simulink library "mbed_lib.tmp"  (R2015a)
settings: Solver=ode45  SolverMode=SingleTasking  StartTime=0.0  StopTime=10.0  RelTol=1e-3
undefined symbols (not defined in the file): A
libraries: mbed_lib x1
settings Model: CovSFcnEnable=off  Creator=syoon  LastModifiedBy=oh
settings OptimizationCC: BlockReduction=off  BooleanDataType=off
settings DebuggingCC: SaveWithParameterizedLinksMsg=none  UnderspecifiedInitializationDetection=Classic  MergeDetectMultiDrivingBlocksExec=none  SignalResolutionControl=TryResolveAllWithWarning  StrictBusMsg=Warning
settings HardwareCC: TargetUnknown=on

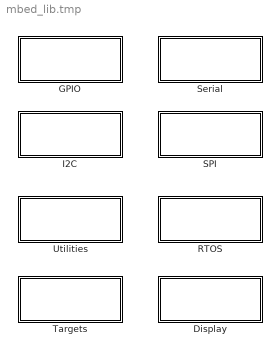
== system mbed_lib.tmp ==
  Display : Subsystem
      settings: OpenFcn=LCDScope
      mask Display: disp('Display')
  GPIO : Subsystem
      mask Display: disp('GPIO')
  I2C : Subsystem
      mask Display: disp('I2C')
  RTOS : Subsystem
      mask Display: disp('RTOS')
  SPI : Subsystem
      mask Display: disp('SPI')
  Serial : Subsystem
      mask Display: disp('Serial')
  Targets : Subsystem
      settings: OpenFcn=mbed_targets
      mask Display: disp('Targets')
  Utilities : Subsystem
      mask Display: disp('Utilities')

== system mbed_lib.tmp/Display ==

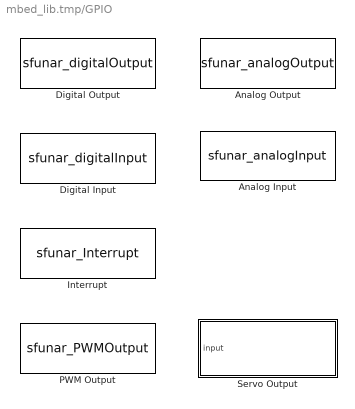
== system mbed_lib.tmp/GPIO ==
  Analog Input : S-Function  FunctionName=sfunar_analogInput  Parameters=uint8(SParameter1), SampleTime, uint8(SParameter2)  mask(mbed Analog Input){SParameter2=A, SParameter1=0, SampleTime=-1}
      mask prompts: SParameter2 "Port Name:"; SParameter1 "Pin Number:"; SampleTime "Sample time (-1 for inherited):"
      mask help:
      | Reads the analog voltage input from the specified pin.
      |
      | The range of input on the pin is between 0 and Vref corresponding to a block output of 0 to 1.0f (in %) or 0 to 1024/4096/.. .
      mask Help:
      | <p>This block calls the AnalogIn.read() and AnalogIn.read_u16() function from the mbed library.
      | <p>For more information see: <a href="http://mbed.org ...">Arduino - AnalogRead</a>
      mask TypeOptions SParameter2: A | B | C | D | E | F | G | H | I | J | K
      mask TypeOptions SParameter1: 0 | 1 | 2 | 3 | 4 | 5 | 6 | 7 | 8 | 9 | 10 | 11 | 12 | 13 | 14 | 15
      mask Display:
      | offset=0.0;
      | plot([0+offset:0.025:0.25+offset],0.3*sin(2*pi*[0:0.1:1])+0.5)
      | disp(['Pin ', SParameter2+64, '.', num2str(SParameter1-1)]);
      | port_label('output',1,'RAW');
      | port_label('output',2,'0-1.0f');
  Analog Output : S-Function  FunctionName=sfunar_analogOutput  Parameters=uint8(SParameter1), SampleTime, uint8(SParameter2), uint8(inputVariant)  mask(mbed Analog Output){SParameter2=A, SParameter1=0, inputVariant=Double: 0 - 1.0f, SampleTime=-1}
      mask prompts: SParameter2 "Port Name:"; SParameter1 "Pin Number:"; inputVariant "Input data format"; SampleTime "Sample time (-1 for inherited):"
      mask help:
      | Writes an analog voltage output to the specified pin using the integrated DAC.
      |
      | The input to this block is a float between 0 and 1.0 (in %) or an integer between 0 and 1024/4096/.. corresponding to an output voltage between 0 to Vref.
      mask Help:
      | <p>This block calls the analogWrite() function from the Arduino language library.
      | <p>For more information see: <a href="http://arduino.cc/en/Reference/AnalogWrite">Arduino - AnalogWrite</a>
      mask TypeOptions SParameter2: A | B | C | D | E | F | G | H | I | J | K
      mask TypeOptions SParameter1: 0 | 1 | 2 | 3 | 4 | 5 | 6 | 7 | 8 | 9 | 10 | 11 | 12 | 13 | 14 | 15
      mask TypeOptions inputVariant: Uint16: RAW (0x0YYY) | Double: 0 - 1.0f
      mask Display:
      | offset=0.7;
      | plot([0+offset:0.025:0.25+offset],0.3*sin(2*pi*[0:0.1:1])+0.5)
      | disp(['Pin ', SParameter2+64, '.', num2str(SParameter1-1)]);
      | p={'RAW'; '0-1.0f'};
      | port_label('input',1,p{inputVariant});
  Digital Input : S-Function  FunctionName=sfunar_digitalInput  Parameters=uint8(SParameter1), SampleTime, uint8(SParameter2), uint8(SParameter3)  mask(mbed Digital Input){SParameter2=A, SParameter1=0, SParameter3=PullDefault, SampleTime=-1}
      mask prompts: SParameter2 "Port Name"; SParameter1 "Pin Number:"; SParameter3 "Input Mode"; SampleTime "Sample time (-1 for inherited):"
      mask help:
      | Reads the digital value from the specified pin.
      |
      | The block outputs 1 for high and 0 for low.
      mask Help:
      | <p>This block uses the DigitalIn api of the mbed library.
      | <p>For more information see: <a href="http://arduino.cc/en/Reference/DigitalRead">Arduino - DigitalRead</a>
      mask TypeOptions SParameter2: A | B | C | D | E | F | G | H | I | J | K
      mask TypeOptions SParameter1: 0 | 1 | 2 | 3 | 4 | 5 | 6 | 7 | 8 | 9 | 10 | 11 | 12 | 13 | 14 | 15
      mask TypeOptions SParameter3: PullDefault | PullUp | PullDown | PullNone
      mask Display:
      | plot([0 0.15 0.15 0.35 0.35 0.5],[0.3 0.3 0.7 0.7 0.3 0.3])
      | port_label('output',1,['Pin ', SParameter2+64, '.', num2str(SParameter1-1)]);
  Digital Output : S-Function  FunctionName=sfunar_digitalOutput  Parameters=uint8(SParameter1), SampleTime, uint8(SParameter2), uint8(SParameter3)  mask(mbed Digital Output){SParameter2=A, SParameter1=0, SParameter3=PullDefault, SampleTime=-1}
      mask prompts: SParameter2 "Port Name:"; SParameter1 "Pin Number:"; SParameter3 "Output Mode"; SampleTime "Sample time (-1 for inherited):"
      mask help:
      | Sends the digital value to the specified port.pin.
      | The pin can be configured as push-pull (pp) or open drain output (od).
      |
      | An input of 1 sets the pin high and 0 sets the pin low.
      mask Help:
      | <p>This block uses the DigitalOut class of the mbed library.
      | <p>For more information see: <a href="http://mbed.org">mbed - DigitalWrite</a>
      mask TypeOptions SParameter2: A | B | C | D | E | F | G | H | I | J | K
      mask TypeOptions SParameter1: 0 | 1 | 2 | 3 | 4 | 5 | 6 | 7 | 8 | 9 | 10 | 11 | 12 | 13 | 14 | 15
      mask TypeOptions SParameter3: PullDefault | PullUp | PullDown | PullNone | Repeater | OpenDrain
      mask Display:
      | plot([0.5 0.65 0.65 0.85 0.85 1],[0.3 0.3 0.7 0.7 0.3 0.3])
      | port_label('input',1,['Pin ', SParameter2+64, '.', num2str(SParameter1-1)]);
  Interrupt : S-Function  FunctionName=sfunar_Interrupt  Parameters=uint8(PortName), uint8(PinName), uint8(Interrupt)  mask{PortName=A, PinName=0, Interrupt=None}
      mask prompts: PortName "Port Name"; PinName "Pin Name"
      mask TypeOptions PortName: A | B | C | D | E | F | G | H | I | J | K
      mask TypeOptions PinName: 0 | 1 | 2 | 3 | 4 | 5 | 6 | 7 | 8 | 9 | 10 | 11 | 12 | 13 | 14 | 15
      mask TypeOptions Interrupt: None | Rise | Fall | Both
      mask Display:
      | p={'None'; 'Rise'; 'Fall'; 'Both'};
      | disp(['Interrupt: ' p{Interrupt} ' Pin ', PortName+64, '.', num2str(PinName-1)]);
  PWM Output : S-Function  FunctionName=sfunar_PWMOutput  Parameters=SampleTime, uint8(SParameter1), uint8(SParameter2), uint32(SParameter3)  mask(mbed PWM Output){SParameter1=A, SParameter2=0, SParameter3=1000, SampleTime=-1}
      mask prompts: SParameter1 "PWM Port:"; SParameter2 "PWM Pin:"; SParameter3 "Period (µs):"; SampleTime "Sample time (-1 for inherited):"
      mask help:
      | Creates an pwm output signal on the specified pin using a configurable PWM period.
      |
      | The input to this block is a float between 0.0f and 1.0f corresponding to 0 to 100% pulsewidth.
      mask Help:
      | <p>This block calls the analogWrite() function from the Arduino language library.
      | <p>For more information see: <a href="http://arduino.cc/en/Reference/AnalogWrite">Arduino - AnalogWrite</a>
      mask TypeOptions SParameter1: A | B | C | D | E | F | G | H | I | J | K
      mask TypeOptions SParameter2: 0 | 1 | 2 | 3 | 4 | 5 | 6 | 7 | 8 | 9 | 10 | 11 | 12 | 13 | 14 | 15
      mask Display:
      | plot([0.5 0.65 0.65 0.85 ],[0.3 0.3 0.7 0.7 ])
      | plot([0.8 0.8],[0.7 0.3])
      | plot([0.825 0.825],[0.7 0.3])
      | plot([0.85 0.85],[0.7 0.3])
      | plot([0.8 1],[0.3 0.3])
      | disp(['Pin ' SParameter1+64 '.' num2str(SParameter2-1)]);
      | port_label('input',1,'0-1.0f');
  Servo Output : Subsystem  mask{SParameter1=A, SParameter2=0, PW_min=1, PW_max=2}
      mask prompts: SParameter1 "PWM Port:"; SParameter2 "PWM Pin:"; PW_min "PW min (ms)"; PW_max "PW max (ms)"
      mask help:
      | Block generates PWM signal with 50Hz period for control of standard RC-servo.
      | Minimum and maximum pulsewidth can be configured.
      | Input is a double value between 0 and 1.0
      mask TypeOptions SParameter1: PWM Output/SParameter1
      mask TypeOptions SParameter2: PWM Output/SParameter2
      mask Display:
      | disp('Servo Output\n');
      | disp(['\nPin ' SParameter1+64 '.' num2str(SParameter2-1) ]);
      | port_label('input',1,'0-1.0f');

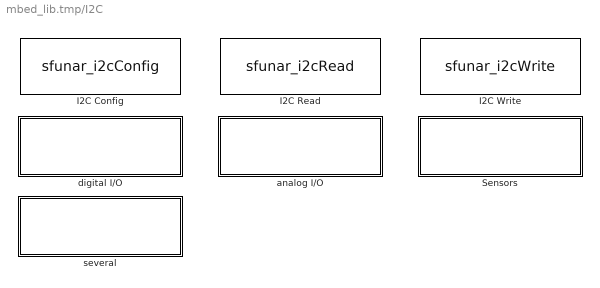
== system mbed_lib.tmp/I2C ==
  I2C Config : S-Function  Priority=0  FunctionName=sfunar_i2cConfig  Parameters=uint8(0), uint8(SParameter2), uint8(SParameter3), uint8(SParameter4), uint8(SParameter5), SParameter6, uint8(I2cPort)  mask(I2C Configuration){I2cPort=1, SParameter6=100000, SParameter2=B, SParameter3=9, SParameter4=B, SParameter5=8}
      mask prompts: I2cPort "I2C Port"; SParameter6 "Bus frequency: [Hz]"; SParameter2 "Port Name (SDA)"; SParameter3 "Pin Number (1-16):"; SParameter4 "Port Name (SCL)"; SParameter5 "Pin Number (1-16):"
      mask help: This block sets up the I2C connection on the mbed board. You must have one of these blocks in any model that ues I2C blocks.
      mask Help: helpview([mbed_getTargetRootPath '/doc/_build/htmlhelp/chapters/I2c_Config_en.html'])
      mask TypeOptions I2cPort: 1 | 2 | 3
      mask TypeOptions SParameter2: A | B | C | D | E | F
      mask TypeOptions SParameter3: 0 | 1 | 2 | 3 | 4 | 5 | 6 | 7 | 8 | 9 | 10 | 11 | 12 | 13 | 14 | 15
      mask TypeOptions SParameter4: A | B | C | D | E | F
      mask TypeOptions SParameter5: 0 | 1 | 2 | 3 | 4 | 5 | 6 | 7 | 8 | 9 | 10 | 11 | 12 | 13 | 14 | 15
      mask Display:
      | disp(['I2C ' num2str(I2cPort) '\n\n']);
      | disp(['SDA: ' SParameter2+64 '.' num2str(SParameter3-1) ', SCL: ' SParameter4+64, '.' num2str(SParameter5-1)]);
      | disp(['\n\nFrequency: ' num2str(SParameter6) ' HZ']);
  I2C Read : S-Function  FunctionName=sfunar_i2cRead  Parameters=SampleTime, boolean(AddressFlag), uint8(SlaveAddress), boolean(ByteCountFlag), uint8(NumBytes), boolean(Repeated), uint8(I2cPort), uint8(AckOut)  mask(I2C Read){I2cPort=1, AddressFlag=off, SlaveAddress=0, ByteCountFlag=off, NumBytes=1, Repeated=off, AckOut=off, SampleTime=-1}
      mask prompts: I2cPort "I2C Port:"; AddressFlag "external address input"; SlaveAddress "Slave address:"; ByteCountFlag "external byte count"; NumBytes "Number of bytes to read:"; AckOut "Enable ACK Ouput"; SampleTime "Sample time (-1 for inherited):"
      mask help:
      | Performs a read operation from the device at the given bus address.
      |
      | data types:
      | data out port   --> uint8
      | address in port --> uint8
      | byte count port --> uint8
      | ack port        --> uint8
      mask Help: helpview([mbed_getTargetRootPath '/doc/_build/htmlhelp/chapters/I2c_Read_en.html'])
      mask TypeOptions I2cPort: 1 | 2 | 3
      mask Display:
      | disp(['I2C ' num2str(I2cPort) '\n']);
      | if AddressFlag == 0
      |     disp(['\nAddress: 0x' dec2hex(SlaveAddress)]);
      | else
      |    disp(['\nAddress: external']);
      |    port_label('input',1,'addr');
      | end
      | 
      | if ByteCountFlag == 1 && AddressFlag == 0
      |     port_label('input',1,'cnt');
      | elseif ByteCountFlag == 1 && AddressFlag == 1
      |     port_label('input',2,'cnt');
      | end
      | 
      | port_label('output',1,'data');
      | if AckOut == 1
      |     port_label('output',2,'ACK');
      | end
  I2C Write : S-Function  FunctionName=sfunar_i2cWrite  Parameters=SampleTime, boolean(AddressFlag), uint8(SlaveAddress), boolean(ByteCountFlag), boolean(Repeated), uint8(I2cPort), uint8(AckOut)  mask(I2C Write){I2cPort=1, AddressFlag=off, SlaveAddress=0, ByteCountFlag=off, Repeated=off, AckOut=off, SampleTime=-1}
      mask prompts: I2cPort "I2C Port:"; AddressFlag "external address input"; SlaveAddress "Slave address:"; ByteCountFlag "external byte count"; AckOut "Enable ACK Output"; SampleTime "Sample time (-1 for inherited):"
      mask help:
      | Performs a write operation to the device at the given bus address.
      |
      | data types:
      | data in port --> uint8
      | address in port --> uint8
      | byte count port --> uint8
      | ack port  --> uint8
      mask Help: helpview([mbed_getTargetRootPath '/doc/_build/htmlhelp/chapters/I2c_Write_en.html'])
      mask TypeOptions I2cPort: 1 | 2 | 3
      mask Display:
      | disp(['I2C ' num2str(I2cPort) '\n']);
      | 
      | port_label('input', 1, 'data');
      | 
      | if AddressFlag == 1
      |     disp(['\nAddress: external']);
      |     port_label('input', 2, 'addr');
      | else
      |     disp(['\nAddress: 0x' dec2hex(SlaveAddress)]);
      | end
      | 
      | if AddressFlag == 0 && ByteCountFlag == 1
      |     port_label('input', 2, 'cnt');
      | elseif AddressFlag == 1 && ByteCountFlag == 1
      |     port_label('input', 3, 'cnt');
      | end
      | 
      | if AckOut == 1
      |     port_label('output',1,'ACK');
      | end
  Sensors : Subsystem
      settings: OpenFcn=mbed_i2c_sensors
  analog I/O : Subsystem
      settings: OpenFcn=mbed_i2c_analog_io
  digital I/O : Subsystem
      settings: OpenFcn=mbed_i2c_digital_io
  several : Subsystem
      settings: OpenFcn=mbed_i2c_several

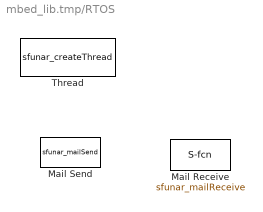
== system mbed_lib.tmp/RTOS ==
  Mail Receive : S-Function  FunctionName=sfunar_mailReceive  Parameters=MailNumber, uint32(DataType), uint32(NumElements)  mask{MailNumber=1, DataType=double, NumElements=1}
      mask prompts: MailNumber "Mail number"; DataType "Data type"; NumElements "Number of output elements"
      mask TypeOptions MailNumber: 1 | 2 | 3 | 4 | 5 | 6 | 7 | 8 | 9
      mask TypeOptions DataType: double | single | int8 | uint8 | int16 | uint16 | int32 | uint32
      mask Display:
      | disp(['Mail ' num2str(MailNumber)]);
      | port_label('output',1,'d');
      | port_label('output',2,'new');
  Mail Send : S-Function  FunctionName=sfunar_mailSend  Parameters=MailNumber, DataType, uint32(NumElements), uint32(Depth)  mask{MailNumber=1, DataType=double, NumElements=1, Depth=1}
      mask prompts: MailNumber "Mail Number"; DataType "Data type"; NumElements "Number of input elements"; Depth "Number of mails in queue"
      mask TypeOptions MailNumber: 1 | 2 | 3 | 4 | 5 | 6 | 7 | 8 | 9
      mask TypeOptions DataType: double | single | int8 | uint8 | int16 | uint16 | int32 | uint32
      mask Display:
      | disp(['Mail ' num2str(MailNumber)]);
      | port_label('input',1,'d');
  Thread : S-Function  FunctionName=sfunar_createThread  Parameters=ThreadPriority, StackOption, uint32(StackSize), uint32(Timing)  mask{ThreadPriority=Normal, Timing=0, StackOption=Default, StackSize=0}
      mask prompts: ThreadPriority "Thread Priority"; StackOption "Stack size"; StackSize "Size:"
      mask TypeOptions ThreadPriority: Idle | Low | Below Normal | Normal | Above Normal | High | Realtime
      mask TypeOptions StackOption: Default | User defined
      mask Display: disp('create RtosThread');

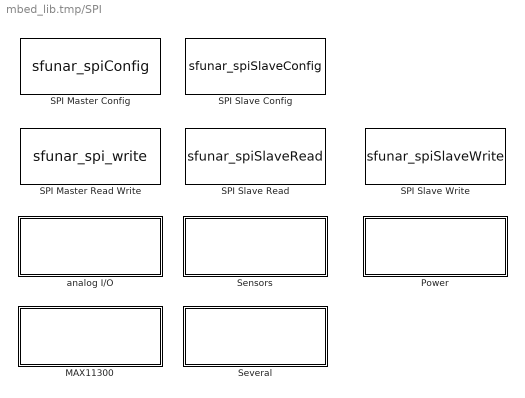
== system mbed_lib.tmp/SPI ==
  MAX11300 : Subsystem
      settings: OpenFcn=mbed_spi_max11300
  Power : Subsystem
      settings: OpenFcn=mbed_spi_power
  SPI Master Config : S-Function  Priority=0  FunctionName=sfunar_spiConfig  Parameters=uint8(0), uint8(MosiPort), uint8(MosiPin), uint8(MisoPort), uint8(MisoPin), SpiFreq, uint8(SclkPort), uint8(SclkPin), uint8(SpiPort)  mask(SPI Configuration){SpiPort=1, SpiFreq=100000, MosiPort=A, MosiPin=7, MisoPort=A, MisoPin=6, SclkPort=A, SclkPin=5}
      mask prompts: SpiPort "SPI Port"; SpiFreq "Bus frequency: [Hz]"; MosiPort "MOSI: Port"; MosiPin "Pin"; MisoPort "MISO: Port"; MisoPin "Pin"; SclkPort "SCLK: Port"; SclkPin "Pin"
      mask help: This block sets up the SPI connection on the mbed board. You must have one of these blocks in any model that ues SPI blocks.
      mask Help: helpview([mbed_getTargetRootPath '/doc/_build/htmlhelp/chapters/Spi_Master_Config_en.html'])
      mask TypeOptions SpiPort: 1 | 2 | 3 | 4
      mask TypeOptions MosiPort: A | B | C | D | E | F | G | H | I | NC
      mask TypeOptions MosiPin: 0 | 1 | 2 | 3 | 4 | 5 | 6 | 7 | 8 | 9 | 10 | 11 | 12 | 13 | 14 | 15
      mask TypeOptions MisoPort: A | B | C | D | E | F | G | H | I | NC
      mask TypeOptions MisoPin: 0 | 1 | 2 | 3 | 4 | 5 | 6 | 7 | 8 | 9 | 10 | 11 | 12 | 13 | 14 | 15
      mask TypeOptions SclkPort: A | B | C | D | E | F | G | H | I
      mask TypeOptions SclkPin: 0 | 1 | 2 | 3 | 4 | 5 | 6 | 7 | 8 | 9 | 10 | 11 | 12 | 13 | 14 | 15
      mask Display:
      | disp(['SPI ' num2str(SpiPort) '\n\n\n']);
      | str1='';
      | if MosiPort==10
      |   str1 = 'NC';
      | else
      |   str1 = ['P' MosiPort+64 '_' num2str(MosiPin-1)];
      | end
      | str2='';
      | if MisoPort==10
      |   str2 = 'NC';
      | else
      |   str2 = ['P' MisoPort+64, '_' num2str(MisoPin-1)];
      | end
      | disp(['\nMOSI: ' str1 ', MISO: ' str2 ' \n\n']);
      | disp(['\n\nSCK: P' SclkPort+64, '_' num2str(SclkPin-1) ' \n']);
      | disp(['\n\n\nFrequency: ' num2str(SpiFreq) ' HZ']);
  SPI Master Read Write : S-Function  FunctionName=sfunar_spi_write  Parameters=SpiPort, CsPort, CsPin  mask(SPI Master Read Write){SpiPort=1, CsPort=A, CsPin=0}
      mask prompts: SpiPort "SPI Port"; CsPort "Chip Select Port"; CsPin "Pin"
      mask help: Perfoms a one byte write operation to the SPI bus and returns the received byte.
      mask Help: helpview([mbed_getTargetRootPath '/doc/_build/htmlhelp/chapters/Spi_Master_Read_Write_en.html'])
      mask TypeOptions SpiPort: 1 | 2 | 3 | 4
      mask TypeOptions CsPort: A | B | C | D | E | F | G | H
      mask TypeOptions CsPin: 0 | 1 | 2 | 3 | 4 | 5 | 6 | 7 | 8 | 9 | 10 | 11 | 12 | 13 | 14 | 15
      mask Display:
      | disp('SPI Master Read/Write\n\n');
      | disp(['SPI ' num2str(SpiPort)]);
      | 
      | disp(['\n\nChip Select: ' CsPort+64 '.' num2str(CsPin-1)]);
  SPI Slave Config : S-Function  FunctionName=sfunar_spiSlaveConfig  Parameters=BusSpeed, MosiPort, MosiPin, MisoPort, MisoPin, SckPort, SckPin, SselPort, SselPin  mask(SPI Slave Config){BusSpeed=100000, MosiPort=A, MosiPin=0, MisoPort=A, MisoPin=0, SckPort=A, SckPin=0, SselPort=A, SselPin=0}
      mask prompts: BusSpeed "Bus frequency: [Hz]"; MosiPort "MOSI: Port"; MosiPin "Pin"; MisoPort "MISO: Port"; MisoPin "Pin"; SckPort "SCK: Port"; SckPin "Pin"; SselPort "SSEL: Port"; SselPin "Pin"
      mask help: This block sets up the SPI connection on the mbed board to act as a slave device to an external master.
      mask Help: helpview([mbed_getTargetRootPath '/doc/_build/htmlhelp/chapters/Spi_Slave_Config_en.html'])
      mask TypeOptions MosiPort: A | B | C | D | E | F
      mask TypeOptions MosiPin: 0 | 1 | 2 | 3 | 4 | 5 | 6 | 7 | 8 | 9 | 10 | 11 | 12 | 13 | 14 | 15
      mask TypeOptions MisoPort: A | B | C | D | E | F
      mask TypeOptions MisoPin: 0 | 1 | 2 | 3 | 4 | 5 | 6 | 7 | 8 | 9 | 10 | 11 | 12 | 13 | 14 | 15
      mask TypeOptions SckPort: A | B | C | D | E | F
      mask TypeOptions SckPin: 0 | 1 | 2 | 3 | 4 | 5 | 6 | 7 | 8 | 9 | 10 | 11 | 12 | 13 | 14 | 15
      mask TypeOptions SselPort: A | B | C | D | E | F
      mask TypeOptions SselPin: 0 | 1 | 2 | 3 | 4 | 5 | 6 | 7 | 8 | 9 | 10 | 11 | 12 | 13 | 14 | 15
      mask Display:
      | disp(['Frequency: ' num2str(BusSpeed) ' HZ\n\n']);
      | disp(['\nMOSI: ' MosiPort+64 '.' num2str(MosiPin-1) ', MISO: ' MisoPort+64, '.' num2str(MisoPin-1) '\n']);
      | disp(['\n\n\nSCK: ' SckPort+64, '.' num2str(SckPin-1) ',SSEL: ' SselPort+64 '.' num2str(SselPin-1) '\n']);
  SPI Slave Read : S-Function  FunctionName=sfunar_spiSlaveRead  Parameters=SampleTime  mask(SPI Slave Read){SampleTime=-1}
      mask prompts: SampleTime "Sampel time: (-1 for inherited)"
      mask help: Reads the last received value from the spi input buffer.
      mask Help: helpview([mbed_getTargetRootPath '/doc/_build/htmlhelp/chapters/Spi_Slave_Read_en.html'])
      mask Display: disp('SPI Slave Read')
  SPI Slave Write : S-Function  FunctionName=sfunar_spiSlaveWrite  Parameters=SampleTime  mask(SPI Slave Write){SampleTime=-1}
      mask prompts: SampleTime "Sample time: (-1 for inherited)"
      mask help: This block puts one byte in the spi output buffer
      mask Help: helpview([mbed_getTargetRootPath '/doc/_build/htmlhelp/chapters/Spi_Slave_Write_en.html'])
      mask Display: disp('SPI Slave Write');
  Sensors : Subsystem
      settings: OpenFcn=mbed_spi_sensors
  Several : Subsystem
      settings: OpenFcn=mbed_spi_several
  analog I/O : Subsystem
      settings: OpenFcn=mbed_spi_analog_io

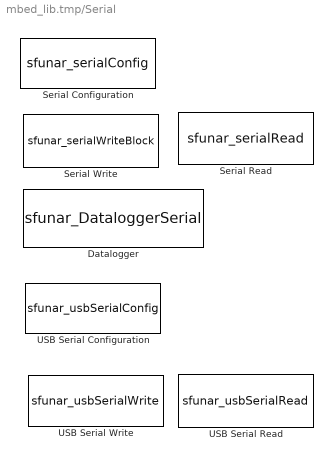
== system mbed_lib.tmp/Serial ==
  Datalogger : S-Function  FunctionName=sfunar_DataloggerSerial  Parameters=uint8(SerialPort), TypeInputPorts, SampleTime, uint8(errEn), uint32(BufferSize)  mask(Write csv style String to choosen Serial Port){SerialPort=1, TypeInputPorts={ 'uint8' 8 'int8' 4 'bool' 1 }, TypeOfInputs={'8*uint8' '4*int8' '1*bool'}, BufferSize=100, errEn=off, SampleTime=-1}
      mask prompts: SerialPort "Serial Port"; TypeInputPorts "Type of Inputs"; TypeOfInputs "Type of Inputs"; BufferSize "Buffer size"; errEn "Enable error output port"; SampleTime "Sample time (-1 for inherited):"
      mask help:
      | Parameters:
      | Serial Port:
      |  select Serial Port - corresponding config block is neccessary
      |
      | Type of Inputs:
      | List of 2-tuples
      |  1. item: Port width
      |  2. item: Port data type (single, double, int8, int16, int32, int64, uint8, uint16, uint32, uint64, bool)
      |  e.g.: {'8*uint8' '4*int8' '1*bool'}
      mask TypeOptions SerialPort: 1 | 2 | 3 | 4 | 5
      mask Callback TypeOfInputs:
      | cfg=eval(get_param(gcb,'TypeOfInputs'));
      | str={};
      | 
      | for i=1:size(cfg,2)
      |     res = strsplit(cfg{i}, '*');
      |     if isempty(str)
      |         str = strjoin({['''' res{2} ''''] res{1}});
      |     else
      |         str = strjoin({str ['''' res{2} ''''] res{1}});
      |     end
      | end
      | str = strjoin({'{' str '}'});
      | 
      | set_param(gcb,'TypeInputPorts', str);
      mask Display:
      | disp(['Datalogger Serial\n\n']);
      | disp(['\n\nSerial ' SerialPort+48]);
      | if errEn
      |     port_label('output',1,'Error');
      | end
      | for i=1:2:size(TypeInputPorts,2)
      |     port_label('input',(i+1)/2, [TypeInputPorts{i} ':' num2str(TypeInputPorts{i+1})]);
      | end
  Serial Configuration : S-Function  FunctionName=sfunar_serialConfig  Parameters=uint8(SerialPort), uint8(TXPort), uint8(TXPin), uint8(RXPort), uint8(RXPin), BaudRate  mask(mbed Serial Configuration){SerialPort=1, TXPort=A, TXPin=2, RXPort=A, RXPin=3, BaudRate=9600}
      mask prompts: SerialPort "Serial Port"; TXPort "Port Name (TX)"; TXPin "Pin Number (1-16):"; RXPort "Port Name (RX)"; RXPin "Pin Number (1-16):"; BaudRate "Baud Rate:"
      mask help:
      | This blocks sets up the serial connection on the mbed board. You must have one of these blocks in any model that ues the Serial Write or Serial Read blocks.
      |
      | Set the baud rate to match the device that you are communicating with. Standard rates include:300, 1200, 2400, 4800, 9600, 14400, 19200, 28800, 38400, 57600, or 115200.
      mask TypeOptions SerialPort: 1 | 2 | 3 | 4 | 5
      mask TypeOptions TXPort: A | B | C | D | E | F
      mask TypeOptions TXPin: 0 | 1 | 2 | 3 | 4 | 5 | 6 | 7 | 8 | 9 | 10 | 11 | 12 | 13 | 14 | 15
      mask TypeOptions RXPort: A | B | C | D | E | F
      mask TypeOptions RXPin: 0 | 1 | 2 | 3 | 4 | 5 | 6 | 7 | 8 | 9 | 10 | 11 | 12 | 13 | 14 | 15
      mask Display: disp(['Serial config\n\n' 'Serial' num2str(SerialPort) '\nTX ' TXPort+64 '.' num2str(TXPin-1) ', RX ' RXPort+64, '.' num2str(RXPin-1)]);
  Serial Read : S-Function  FunctionName=sfunar_serialRead  Parameters=SampleTime, uint8(SParameter1)  mask(mbed Serial Read){SParameter1=1, SampleTime=-1}
      mask prompts: SParameter1 "Serial Port"; SampleTime "Sample time (-1 for inherited):"
      mask help:
      | Reads one byte from the serial port on the mbed board.
      |
      | Outputs -1 if no data is available to be read.
      mask TypeOptions SParameter1: 1 | 2 | 3 | 4 | 5
      mask Display:
      | p={'Serial1'; 'Serial2'; 'Serial3'; 'Serial4'; 'Serial5'};
      | disp(['Read Block\n\n' p{SParameter1}])
  Serial Write : S-Function  FunctionName=sfunar_serialWriteBlock  Parameters=SampleTime, uint8(SerialPort), uint8(numData)  mask(mbed Serial Write){SerialPort=1, numData=on, SampleTime=-1}
      mask prompts: SerialPort "Serial Port"; numData "Enable datasize Port"; SampleTime "Sample time (-1 for inherited):"
      mask help: Writes the one dimensional vector of uint8 at input port d to the serial port on the mbed board. The length of the vector can be dynamically submitted at input port n or is statically read from input port d configuration.
      mask TypeOptions SerialPort: 1 | 2 | 3 | 4 | 5
      mask Display:
      | p={'Serial1'; 'Serial2'; 'Serial3'; 'Serial4'; 'Serial5'};
      | disp(['Write Block\n\n' p{SerialPort}])
      | port_label('input',1,'d');
      | if numData
      |     port_label('input',2,'n');
      | end
  USB Serial Configuration : S-Function  FunctionName=sfunar_usbSerialConfig  mask(Virtual COM Port USB Device){}
      mask help: This block sets up a virtual COM port via the native USB interface of the micro controller
      mask Display: disp(['USB Serial']);
  USB Serial Read : S-Function  FunctionName=sfunar_usbSerialRead  Parameters=SampleTime, int32(PortWidth)  mask{PortWidth=1, SampleTime=-1}
      mask prompts: PortWidth "specify output port width"; SampleTime "Sample time (-1 for inherited):"
      mask Display:
      | disp('USB Serial Read');
      | port_label('output',1,'d');
      | port_label('output',2,'n');
  USB Serial Write : S-Function  FunctionName=sfunar_usbSerialWrite  Parameters=SampleTime, numData  mask(mbed USB Serial Write){numData=on, SampleTime=-1}
      mask prompts: numData "Enable datasize port"; SampleTime "Sample time (-1 for inherited):"
      mask help: Writes the one dimensional vector of uint8 at input port d to the serial port on the mbed board. The length of the vector can be dynamically submitted at input port n or is statically read from input port d configuration.
      mask Display:
      | disp('USB Serial Write');
      | if numData == 1
      |     port_label('input',1,'d');
      |     port_label('input',2,'n');
      | end

== system mbed_lib.tmp/Targets ==

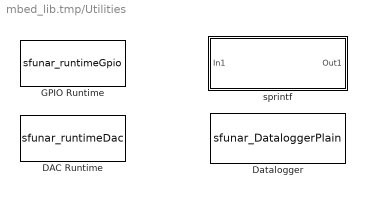
== system mbed_lib.tmp/Utilities ==
  DAC Runtime : S-Function  FunctionName=sfunar_runtimeDac  Parameters=SampleTime, PortName, PinNumber, DacValue  mask(DAC Runtime){PortName=A, PinNumber=0, DacValue=0, SampleTime=-1}
      mask prompts: PortName "Port Name"; PinNumber "Pin Number"; DacValue "DAC Value (0-1.0f)"; SampleTime "Sample time (-1 for inherited)"
      mask help:
      | Sets the DAC output to the configured value when entering the system that contains the block and resets the value after executing the systems code.
      | Can be used for time measurement of multiple subsystems, especially in multitasking models, using only one pin.
      | Setting each block to another DAC value and using an oscilloscope to differentiate between each subsystem.
      mask Help: helpview([mbed_getTargetRootPath '/doc/_build/htmlhelp/chapters/Dac_Runtime_en.html'])
      mask TypeOptions PortName: A | B | C | D | E | F | G | H | I | J
      mask TypeOptions PinNumber: 0 | 1 | 2 | 3 | 4 | 5 | 6 | 7 | 8 | 9 | 10 | 11 | 12 | 13 | 14 | 15
      mask Display:
      | disp('Runtime \nDAC Toggle\n');
      | disp(['\n\nPin ', PortName+64, '.', num2str(PinNumber-1) '  Value: ' num2str(DacValue) ]);
  Datalogger : S-Function  FunctionName=sfunar_DataloggerPlain  Parameters=TypeInputPorts, SampleTime, uint8(errEn), uint32(BufferSize)  mask(Creates a csv style string){TypeInputPorts={ 'uint8' 8 'int8' 4 'bool' 1 }, TypeOfInputs={'8*uint8' '4*int8' '1*bool'}, BufferSize=100, errEn=off, SampleTime=-1}
      mask prompts: TypeInputPorts "Type of Inputs"; TypeOfInputs "Type of Inputs"; BufferSize "Buffer Size"; errEn "Enable error output port"; SampleTime "Sample time (-1 for inherited):"
      mask help:
      | Type of Inputs:
      | List of 2-tuples
      |  1. item: Port width
      |  2. item: Port data type (single, double, int8, int16, int32, int64, uint8, uint16, uint32, uint64, bool)
      |  e.g.: {'8*uint8' '4*int8' '1*bool'}
      |
      | Buffer Size:
      | Estimated maximal size of one data line.
      mask Callback TypeOfInputs:
      | cfg=eval(get_param(gcb,'TypeOfInputs'));
      | str={};
      | 
      | for i=1:size(cfg,2)
      |     res = strsplit(cfg{i}, '*');
      |     if isempty(str)
      |         str = strjoin({['''' res{2} ''''] res{1}});
      |     else
      |         str = strjoin({str ['''' res{2} ''''] res{1}});
      |     end
      | end
      | str = strjoin({'{' str '}'});
      | 
      | set_param(gcb,'TypeInputPorts', str);
      mask Display:
      | disp(['Datalogger']);
      | for i=1:2:size(TypeInputPorts,2)
      |     port_label('input',(i+1)/2, [TypeInputPorts{i} ':' num2str(TypeInputPorts{i+1})]);
      | end
      | port_label('output',1,'d');
      | port_label('output',2,'n');
      | if errEn
      |     port_label('output',3,'Error');
      | end
  GPIO Runtime : S-Function  FunctionName=sfunar_runtimeGpio  Parameters=SampleTime, PortName, PinNumber  mask(GPIO Runtime){PortName=A, PinNumber=0, SampleTime=-1}
      mask prompts: PortName "Port Name"; PinNumber "Pin Number"; SampleTime "Sample time (-1 for inherited)"
      mask help: Toggels a GPIO Pin so that the pulsewidth corresponds to the computational time of the containing subsystem.
      mask Help: helpview([mbed_getTargetRootPath '/doc/_build/htmlhelp/chapters/Gpio_Runtime_en.html'])
      mask TypeOptions PortName: A | B | C | D | E | F | G | H | I | J
      mask TypeOptions PinNumber: 0 | 1 | 2 | 3 | 4 | 5 | 6 | 7 | 8 | 9 | 10 | 11 | 12 | 13 | 14 | 15
      mask Display:
      | disp('Runtime \nGPIO Toggle\n');
      | disp(['\n\nPin ', PortName+64, '.', num2str(PinNumber-1)]);
  sprintf : Subsystem  mask{format=%f\r\n}
      mask TypeOptions format: %f\r\n | %d\r\n | %f | %d
      mask Display:
      | p={'%f\r\n'; '%d\r\n'; '%f'; '%d'};
      | disp(['sprintf: ' p{format}])

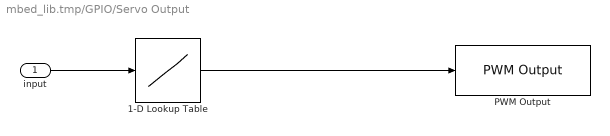
== system mbed_lib.tmp/GPIO/Servo Output ==
  input : Inport
  1-D Lookup Table : Lookup_n-D  NumberOfTableDimensions=1  BreakpointsForDimension1=[0 1]  Table=[PW_min PW_max]/20  ExtrapMethod=Clip  UseLastTableValue=on  InternalRulePriority=Speed  RndMeth=Simplest  InputSameDT=on
  PWM Output : mbed_lib/GPIO/PWM Output  SParameter1=A  SParameter2=0  SParameter3=20000  SampleTime=-1
  wires:
  input/1 -> 1-D Lookup Table/1
  1-D Lookup Table/1 -> PWM Output/1

== system mbed_lib.tmp/I2C/Sensors ==

== system mbed_lib.tmp/I2C/analog I//O ==

== system mbed_lib.tmp/I2C/digital I//O ==

== system mbed_lib.tmp/I2C/several ==

== system mbed_lib.tmp/SPI/MAX11300 ==

== system mbed_lib.tmp/SPI/Power ==

== system mbed_lib.tmp/SPI/Sensors ==

== system mbed_lib.tmp/SPI/Several ==

== system mbed_lib.tmp/SPI/analog I//O ==

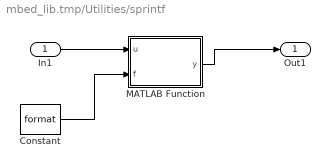
== system mbed_lib.tmp/Utilities/sprintf ==
  In1 : Inport
  Constant : Constant  Value=format
  MATLAB Function : MATLAB Function  TreatAsAtomicUnit=on
  Out1 : Outport
  wires:
  In1/1 -> MATLAB Function/1(u)
  MATLAB Function/1(y) -> Out1/1
  Constant/1 -> MATLAB Function/2(f)

== matlab function mbed_lib.tmp/Utilities/sprintf/MATLAB Function ==
  data: u input; y output; f input
function y = fcn(u,f)
buffer = char(zeros(1,15));
% geht mit 2012b noch nicht aber mit 2014a oder 2013: coder.cinclude('stdio.h');
coder.ceval('#ifdef _WIN32 //');
  if f == 1
    coder.ceval('_snprintf', coder.ref(buffer(int32(1))),int32(size(buffer,2)), ['%f' char(13) char(10) 0], u);
  elseif f == 2
    coder.ceval('_snprintf', coder.ref(buffer(int32(1))),int32(size(buffer,2)), ['%d' char(13) char(10) 0], u);
  elseif f == 3
    coder.ceval('_snprintf', coder.ref(buffer(int32(1))),int32(size(buffer,2)), ['%f' 0], u);
  elseif f == 4
    coder.ceval('_snprintf', coder.ref(buffer(int32(1))),int32(size(buffer,2)), ['%d' 0], u);
  end
coder.ceval('#else //');
  if f == 1
    coder.ceval('snprintf', coder.ref(buffer(int32(1))),int32(size(buffer,2)), ['%f' char(13) char(10) 0], u);
  elseif f == 2
    coder.ceval('snprintf', coder.ref(buffer(int32(1))),int32(size(buffer,2)), ['%d' char(13) char(10) 0], u);
  elseif f == 3
    coder.ceval('snprintf', coder.ref(buffer(int32(1))),int32(size(buffer,2)), ['%f' 0], u);
  elseif f == 4
    coder.ceval('snprintf', coder.ref(buffer(int32(1))),int32(size(buffer,2)), ['%d' 0], u);
  end
coder.ceval('#endif //');
y = uint8(buffer);
